simulink model "unoptimised"  (R2024b)
settings: Solver=VariableStepAuto  StartTime=0.0  StopTime=10  RelTol=1e-3
undefined symbols (not defined in the file or in its folder): b
settings Model: Creator=adubu  LastModifiedBy=adubu
settings OptimizationCC: BlockReduction=off  ConditionallyExecuteInputs=off  DefaultParameterBehavior=Inlined
settings DebuggingCC: AlgebraicLoopMsg=error
settings HardwareCC: ProdBitPerPointer=32  ProdBitPerSizeT=32  ProdBitPerPtrDiffT=32  ProdLargestAtomicFloat=None  ProdIntDivRoundTo=Undefined  ProdEndianess=Unspecified  ProdWordSize=32  ProdHWDeviceType=ASIC/FPGA->ASIC/FPGA  TargetBitPerPointer=64  TargetBitPerSizeT=64  TargetBitPerPtrDiffT=64  TargetLongLongMode=on  TargetIntDivRoundTo=Zero  TargetEndianess=LittleEndian  TargetWordSize=64  TargetHWDeviceType=Custom Processor->MATLAB Host Computer  ProdEqTarget=off

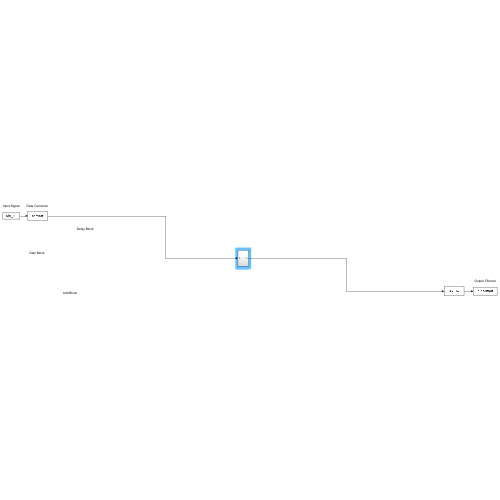
[thumbnail: Simulink's stored preview of the top-level diagram]
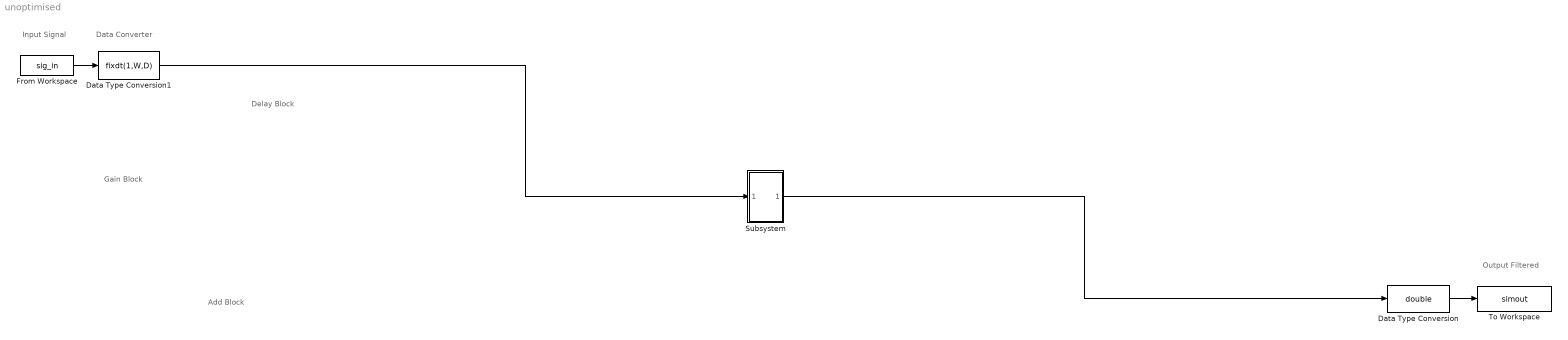
== system unoptimised ==
  note: Input Signal
  note: Data Converter
  note: Delay Block
  note: Gain Block
  note: Add Block
  note: Output Filtered
  Data Type Conversion : DataTypeConversion  OutDataTypeStr=double  SaturateOnIntegerOverflow=off  RndMeth=Floor
  Data Type Conversion1 : DataTypeConversion  OutDataTypeStr=fixdt(1,W,D)  SaturateOnIntegerOverflow=off  RndMeth=Floor
  From Workspace : FromWorkspace  VariableName=sig_in  SampleTime=1  Interpolate=off  ZeroCross=off  OutputAfterFinalValue=Setting to zero
  Subsystem : Subsystem
  To Workspace : ToWorkspace  VariableName=simout  SampleTime=-1
  wires:
  Data Type Conversion/1 -> To Workspace/1
  From Workspace/1 -> Data Type Conversion1/1
  Data Type Conversion1/1 -> Subsystem/1(In1)
  Subsystem/1(Out1) -> Data Type Conversion/1

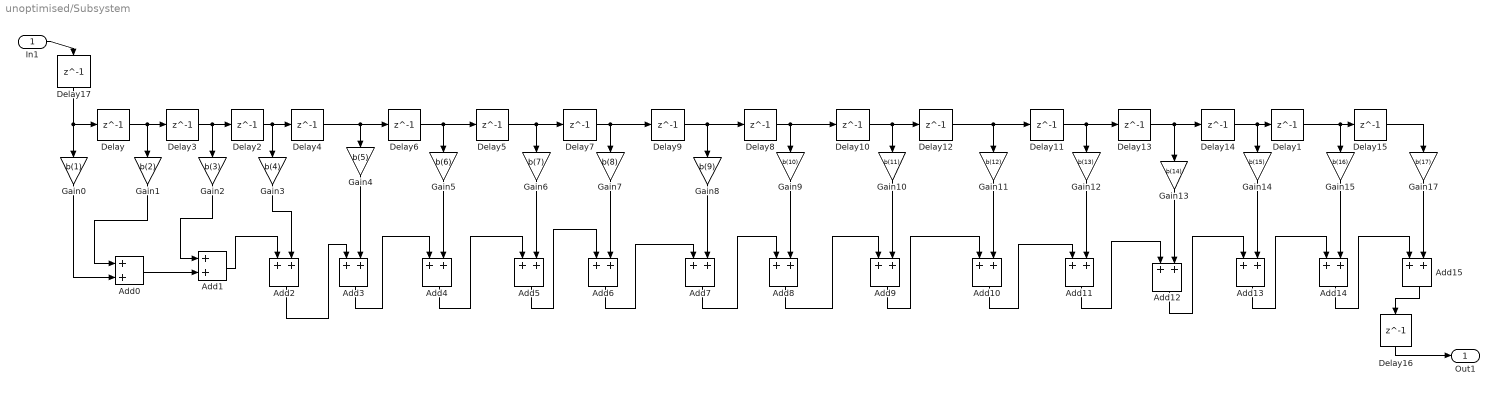
== system unoptimised/Subsystem ==
  In1 : Inport
  Add{0..15} (16 alike) : Sum  OutDataTypeStr=fixdt(1,W,D)  AccumDataTypeStr=fixdt(1,W,D)
  Delay{,1..17} (18 alike) : Delay  DelayLength=1
  Gain0 : Gain  Gain=b(1)  ParamDataTypeStr=fixdt(1,Wg,Dg)  OutDataTypeStr=fixdt(1,Wc,Dc)
  Gain1 : Gain  Gain=b(2)  ParamDataTypeStr=fixdt(1,Wg,Dg)  OutDataTypeStr=fixdt(1,Wc,Dc)
  Gain10 : Gain  Gain=b(11)  ParamDataTypeStr=fixdt(1,Wg,Dg)  OutDataTypeStr=fixdt(1,Wc,Dc)
  Gain11 : Gain  Gain=b(12)  ParamDataTypeStr=fixdt(1,Wg,Dg)  OutDataTypeStr=fixdt(1,Wc,Dc)
  Gain12 : Gain  Gain=b(13)  ParamDataTypeStr=fixdt(1,Wg,Dg)  OutDataTypeStr=fixdt(1,Wc,Dc)
  Gain13 : Gain  Gain=b(14)  ParamDataTypeStr=fixdt(1,Wg,Dg)  OutDataTypeStr=fixdt(1,Wc,Dc)
  Gain14 : Gain  Gain=b(15)  ParamDataTypeStr=fixdt(1,Wg,Dg)  OutDataTypeStr=fixdt(1,Wc,Dc)
  Gain15 : Gain  Gain=b(16)  ParamDataTypeStr=fixdt(1,Wg,Dg)  OutDataTypeStr=fixdt(1,Wc,Dc)
  Gain17 : Gain  Gain=b(17)  ParamDataTypeStr=fixdt(1,Wg,Dg)  OutDataTypeStr=fixdt(1,Wc,Dc)
  Gain2 : Gain  Gain=b(3)  ParamDataTypeStr=fixdt(1,Wg,Dg)  OutDataTypeStr=fixdt(1,Wc,Dc)
  Gain3 : Gain  Gain=b(4)  ParamDataTypeStr=fixdt(1,Wg,Dg)  OutDataTypeStr=fixdt(1,Wc,Dc)
  Gain4 : Gain  Gain=b(5)  ParamDataTypeStr=fixdt(1,Wg,Dg)  OutDataTypeStr=fixdt(1,Wc,Dc)
  Gain5 : Gain  Gain=b(6)  ParamDataTypeStr=fixdt(1,Wg,Dg)  OutDataTypeStr=fixdt(1,Wc,Dc)
  Gain6 : Gain  Gain=b(7)  ParamDataTypeStr=fixdt(1,Wg,Dg)  OutDataTypeStr=fixdt(1,Wc,Dc)
  Gain7 : Gain  Gain=b(8)  ParamDataTypeStr=fixdt(1,Wg,Dg)  OutDataTypeStr=fixdt(1,Wc,Dc)
  Gain8 : Gain  Gain=b(9)  ParamDataTypeStr=fixdt(1,Wg,Dg)  OutDataTypeStr=fixdt(1,Wc,Dc)
  Gain9 : Gain  Gain=b(10)  ParamDataTypeStr=fixdt(1,Wg,Dg)  OutDataTypeStr=fixdt(1,Wc,Dc)
  Out1 : Outport
  wires:
  Add12/1 -> Add13/1
  Delay4/1 -> Gain4/1, Delay6/1
  Delay1/1 -> Delay15/1, Gain15/1
  Gain4/1 -> Add3/2
  Delay6/1 -> Gain5/1, Delay5/1
  Add14/1 -> Add15/1
  Gain9/1 -> Add8/2
  Gain14/1 -> Add13/2
  Gain6/1 -> Add5/2
  Delay/1 -> Gain1/1, Delay3/1
  Delay2/1 -> Gain3/1, Delay4/1
  Gain12/1 -> Add11/2
  Delay5/1 -> Gain6/1, Delay7/1
  Delay13/1 -> Gain13/1, Delay14/1
  Add7/1 -> Add8/1
  Gain0/1 -> Add0/2
  Add8/1 -> Add9/1
  Gain11/1 -> Add10/2
  Gain17/1 -> Add15/2
  Delay10/1 -> Gain10/1, Delay12/1
  Gain8/1 -> Add7/2
  Delay15/1 -> Gain17/1
  Delay12/1 -> Gain11/1, Delay11/1
  Delay7/1 -> Delay9/1, Gain7/1
  Add10/1 -> Add11/1
  Delay3/1 -> Gain2/1, Delay2/1
  Gain5/1 -> Add4/2
  Delay14/1 -> Gain14/1, Delay1/1
  Add0/1 -> Add1/2
  Add6/1 -> Add7/1
  Add5/1 -> Add6/1
  Gain7/1 -> Add6/2
  Add3/1 -> Add4/1
  Gain2/1 -> Add1/1
  Delay9/1 -> Delay8/1, Gain8/1
  Delay11/1 -> Gain12/1, Delay13/1
  Add4/1 -> Add5/1
  Add1/1 -> Add2/1
  Gain1/1 -> Add0/1
  Delay8/1 -> Delay10/1, Gain9/1
  Add11/1 -> Add12/1
  In1/1 -> Delay17/1
  Add2/1 -> Add3/1
  Gain15/1 -> Add14/2
  Add13/1 -> Add14/1
  Gain10/1 -> Add9/2
  Add9/1 -> Add10/1
  Gain3/1 -> Add2/2
  Gain13/1 -> Add12/2
  Add15/1 -> Delay16/1
  Delay17/1 -> Gain0/1, Delay/1
  Delay16/1 -> Out1/1
